simulink model "suspension_model"  (R2023b)
settings: Solver=VariableStepAuto  StartTime=0.0  StopTime=10.0  RelTol=1e-3
undefined symbols (not defined in the file): C, h_0, h_bump, K, m, T, t_bump
libraries: simulink x1
settings Model: Creator=micha  LastModifiedBy=micha

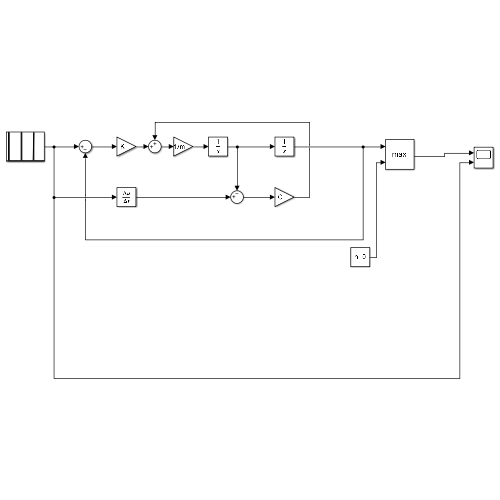
[thumbnail: Simulink's stored preview of the top-level diagram]
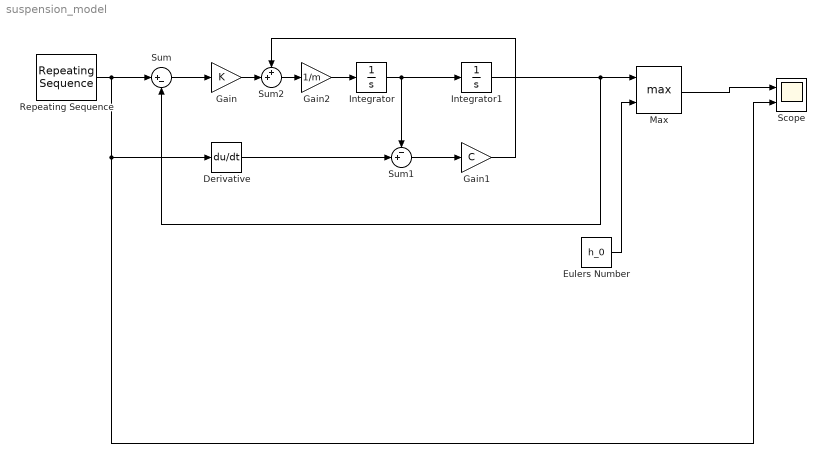
== system suspension_model ==
  Derivative : Derivative
  Eulers Number : Constant  Value=h_0  OutDataTypeStr=Inherit: Inherit via back propagation
  Gain : Gain  Gain=K
  Gain1 : Gain  Gain=C
  Gain2 : Gain  Gain=1/m
  Integrator : Integrator
  Integrator1 : Integrator
  Max : MinMax  Function=max  Inputs=2
  Repeating Sequence : simulink/Sources/Repeating Sequence  rep_seq_t="[0 2 2+t_bump*0.2  2+t_bump*0.8 2+t_bump T]"  rep_seq_y=[h_0 h_0 h_bump h_bump h_0 0]
  Scope : Scope  NumInputPorts=2
  Sum : Sum  Inputs=|+-
  Sum1 : Sum  Inputs=-+|
  Sum2 : Sum  Inputs=++|
  wires:
  Repeating Sequence/1 -> Scope/2, Derivative/1, Sum/1
  Max/1 -> Scope/1
  Eulers Number/1 -> Max/2
  Integrator/1 -> Integrator1/1, Sum1/1
  Integrator1/1 -> Max/1, Sum/2
  Sum/1 -> Gain/1
  Sum1/1 -> Gain1/1
  Sum2/1 -> Gain2/1
  Gain/1 -> Sum2/2
  Gain1/1 -> Sum2/1
  Gain2/1 -> Integrator/1
  Derivative/1 -> Sum1/2
